simulink model "unicycle"  (R2025b)
settings: Solver=VariableStepAuto  StartTime=0.0  StopTime=10.0  RelTol=1e-3
settings Model: Creator=nyanklc  LastModifiedBy=nyanklc

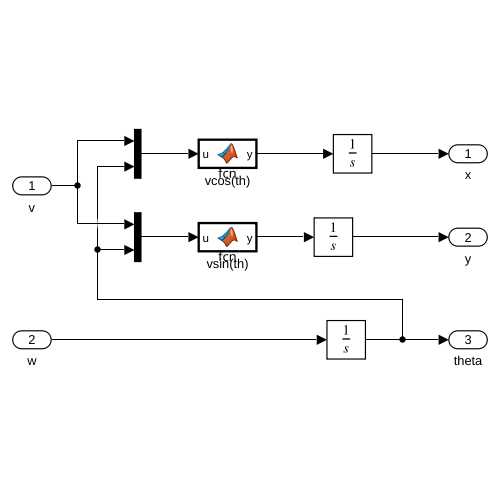
[thumbnail: Simulink's stored preview of the top-level diagram]
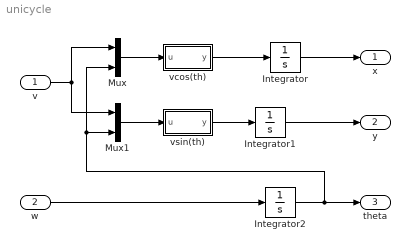
== system unicycle ==
  v : Inport
  w : Inport  Port=2
  Integrator : Integrator
  Integrator1 : Integrator
  Integrator2 : Integrator
  Mux : Mux  Inputs=2
  Mux1 : Mux  Inputs=2
  vcos(th) : MATLAB Function  TreatAsAtomicUnit=on
  vsin(th) : MATLAB Function  TreatAsAtomicUnit=on
  x : Outport
  y : Outport  Port=2
  theta : Outport  Port=3
  wires:
  Integrator/1 -> x/1
  Integrator1/1 -> y/1
  Integrator2/1 -> Mux/2, Mux1/2, theta/1
  w/1 -> Integrator2/1
  vcos(th)/1(y) -> Integrator/1
  Mux/1 -> vcos(th)/1(u)
  v/1 -> Mux1/1, Mux/1
  vsin(th)/1(y) -> Integrator1/1
  Mux1/1 -> vsin(th)/1(u)

== matlab function unicycle/vcos(th) ==
  data: u input; y output
function y = fcn(u)
v = u(1);
theta = u(2);
y = v * cos(theta);

== matlab function unicycle/vsin(th) ==
  data: u input; y output
function y = fcn(u)
v = u(1);
theta = u(2);
y = v * sin(theta);
